simulink subsystem "Day3_Scenario_2"  (R2024a)
settings: Solver=VariableStepAuto  StartTime=0.0  StopTime=10.0  RelTol=1e-3
libraries: CarMaker4SL x8, slpidlib x1
settings Model: Creator=junhyung.cha  LastModifiedBy=User

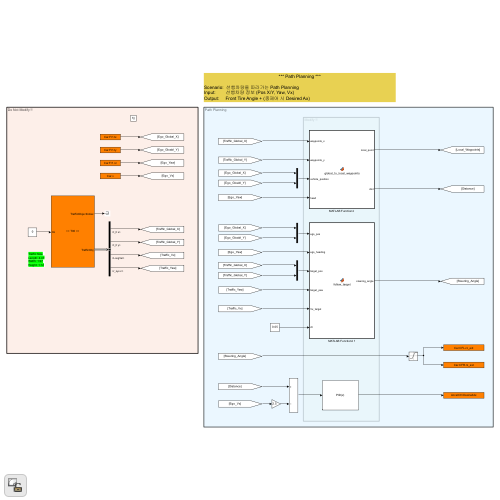
[thumbnail: Simulink's stored preview of the top-level diagram]
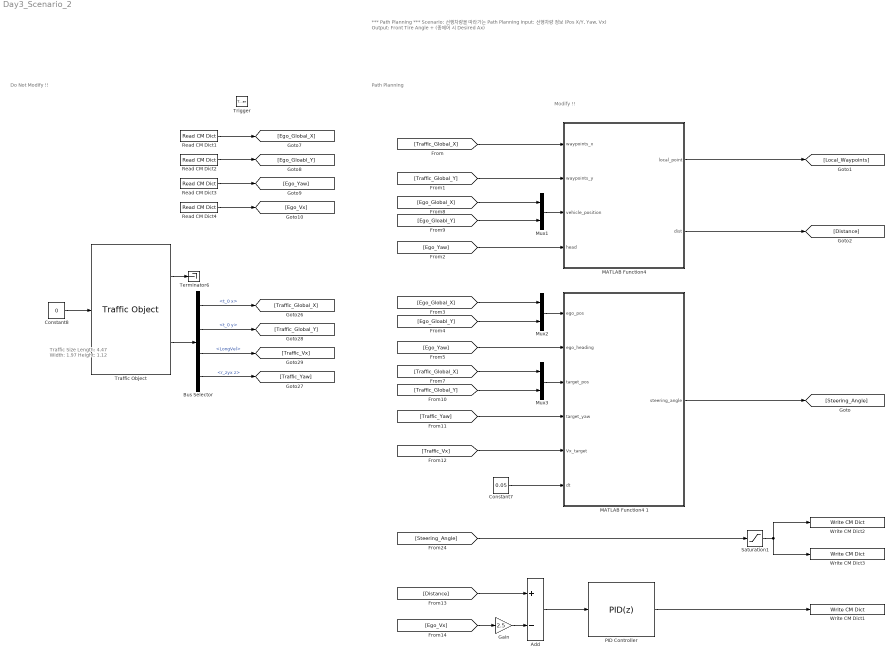
== system Day3_Scenario_2 ==
  note: Path Planning
  note: Do Not Modify !!
  note: Modify !!
  note: *** Path Planning ***
      |
      | Scenario: 선행차량을 따라가는 Path Planning
      | Input: 선행차량 정보 (Pos X/Y, Yaw, Vx)
      | Output: Front Tire Angle + (종제어 시 Desired Ax)
  note: Traffic Size
      | Length: 4.47
      | Width: 1.97
      | Height: 1.12
  Trigger : TriggerPort  TriggerType=function-call  VariantControl=(inherit)
  Add : Sum  Inputs=+-
  Bus Selector : BusSelector  OutputSignals=t_0 x,t_0 y,LongVel,r_zyx z
  Constant7 : Constant  Value=0.05
  Constant8 : Constant  Value=0
  Gain : Gain  Gain=2.5
  "MATLAB Function4 " : MATLAB Function  TreatAsAtomicUnit=on
  MATLAB Function4 1 : MATLAB Function  TreatAsAtomicUnit=on
  Mux1 : Mux  Inputs=2
  Mux2 : Mux  Inputs=2
  Mux3 : Mux  Inputs=2
  PID Controller : slpidlib/PID Controller  Controller=PID  Form=Parallel  TimeDomain=Discrete-time  UseExternalTs=off  SampleTime=-1  IntegratorMethod=Forward Euler  FilterMethod=Forward Euler  ControllerParametersSource=internal  P=3  I=0.01  UseKiTs=off  D=0  UseExternalDerivativeSource=off  N=100  UseFilter=on  TunerSelectOption=Transfer Function Based (PID Tuner App)  InitialConditionSource=internal  InitialConditionForIntegrator=0  InitialConditionForFilter=0  DifferentiatorICPrevScaledInput=0  ExternalReset=none  TrackingMode=off  Kt=1  LimitOutput=off  SatLimitsSource=internal  UpperSaturationLimit=inf  LowerSaturationLimit=-inf  LinearizeAsGain=on  AntiWindupMode=none  Kb=1  LimitIntegrator=off  UpperIntegratorSaturationLimit=inf  LowerIntegratorSaturationLimit=-inf  POutMin=[]  POutMax=[]  IOutMin=[]  IOutMax=[]  DOutMin=[]  DOutMax=[]  NOutMin=[]  NOutMax=[]  SumOutMin=[]  SumOutMax=[]  SaturationOutMin=[]  SaturationOutMax=[]  PParamMin=[]  PParamMax=[]  IParamMin=[]  IParamMax=[]  DParamMin=[]  DParamMax=[]  NParamMin=[]  NParamMax=[]  KbParamMin=[]  KbParamMax=[]  KtParamMin=[]  KtParamMax=[]  KbOutMin=[]  KbOutMax=[]  KtOutMin=[]  KtOutMax=[]  IntegratorOutMin=[]  IntegratorOutMax=[]  FilterOutMin=[]  FilterOutMax=[]  SumI1OutMin=[]  SumI1OutMax=[]  SumI2OutMin=[]  SumI2OutMax=[]  SumI3OutMin=[]  SumI3OutMax=[]  SumI4OutMin=[]  SumI4OutMax=[]  SumDOutMin=[]  SumDOutMax=[]  DifferentiatorOutMin=[]  DifferentiatorOutMax=[]  FilterDiffOutCoefMin=[]  FilterDiffOutCoefMax=[]  ReciprocalOutMin=[]  ReciprocalOutMax=[]  SumDenOutMin=[]  SumDenOutMax=[]  SumNumOutMin=[]  SumNumOutMax=[]  DivideOutMin=[]  DivideOutMax=[]  UdiffTsProdOutMin=[]  UdiffTsProdOutMax=[]  NTsProdOutMin=[]  NTsProdOutMax=[]  UintegralTsProdOutMin=[]  UintegralTsProdOutMax=[]  UngainTsProdOutMin=[]  UngainTsProdOutMax=[]  ClampingZeroOutDataTypeStr=Inherit: Inherit via back propagation  ClampingZeroOutMin=[]  ClampingZeroOutMax=[]  FilterDenConstantOutDataTypeStr=Inherit: Inherit via back propagation  FilterDenConstantOutMin=[]  FilterDenConstantOutMax=[]  PCopyOutDataTypeStr=Inherit: Inherit via back propagation  PCopyOutMin=[]  PCopyOutMax=[]  NCopyOutDataTypeStr=Inherit: Inherit via back propagation  NCopyOutMin=[]  NCopyOutMax=[]  IntegratorContinuousStateAttributes=''  IntegratorStateMustResolveToSignalObject=off  IntegratorRTWStateStorageClass=Auto  FilterContinuousStateAttributes=''  FilterStateMustResolveToSignalObject=off  FilterRTWStateStorageClass=Auto  ParallelPVariant=InternalParameters  IdealPVariant=Disabled  IVariant=InternalParameters  DVariant=InternalParameters  IntegratorVariant=Discrete  SatVariant=Disabled  AWVariant=Passthrough  PCopyVariant=Disabled  TRVariant=Disabled  FdbkBlocksVariant=Forward  IdealPFdbkVariant=Disabled  SatFdbkVariant=Disabled  DerivativeFilterVariant=ForwardEulerFilter  NVariant=InternalParameters  NCopyVariant=Disabled  FilterICVariant=InternalICsFilter  IntegratorICVariant=InternalICs  ExternalResetVariant=Disabled  TRSumVariant=Passthrough  SumFdbkVariant=Disabled  SumVariant=Sum_PID  TsampFilterVariant=InternalTs  TsampNgainVariant=Passthrough  TsampIntegralVariant=Disabled_SignalSpec  ExternalSaturationOutDataTypeStr=Inherit: Same as second input  DerivativeSourceVariant=ErrorSignal
  Read CM Dict1 : CarMaker4SL/Read CM Dict  xname=Car.Fr1.tx  xsync=off  xstime=Inherited
  Read CM Dict2 : CarMaker4SL/Read CM Dict  xname=Car.Fr1.ty  xsync=off  xstime=Inherited
  Read CM Dict3 : CarMaker4SL/Read CM Dict  xname=Car.Fr1.rz  xsync=off  xstime=Inherited
  Read CM Dict4 : CarMaker4SL/Read CM Dict  xname=Car.v  xsync=off  xstime=Inherited
  Saturation1 : Saturate  UpperLimit=pi/6  LowerLimit=-pi/6
  Terminator6 : Terminator
  Traffic Object : CarMaker4SL/Traffic Object  xname=T00  ximode=Traffic Id  xstime=Inherited
      settings: SourceProductName=CarMaker4SL
  Write CM Dict1 : CarMaker4SL/Write CM Dict  xname=AccelCtrl.DesiredAx  xsync=off
  Write CM Dict2 : CarMaker4SL/Write CM Dict  xname=Car.CFL.rz_ext  xsync=off
  Write CM Dict3 : CarMaker4SL/Write CM Dict  xname=Car.CFR.rz_ext  xsync=off
  wires:
  Read CM Dict4/1 -> [Ego_Vx]
  Saturation1/1 -> Write CM Dict3/1, Write CM Dict2/1
  Read CM Dict3/1 -> [Ego_Yaw]
  Read CM Dict1/1 -> [Ego_Global_X]
  Read CM Dict2/1 -> [Ego_Gloabl_Y]
  [Steering_Angle] -> Saturation1/1
  Traffic Object/2 -> Bus Selector/1
  Constant8/1 -> Traffic Object/1
  Bus Selector/4 -> [Traffic_Yaw]  "<r_zyx z>"
  Bus Selector/3 -> [Traffic_Vx]  "<LongVel>"
  Traffic Object/1 -> Terminator6/1
  Bus Selector/2 -> [Traffic_Global_Y]  "<t_0 y>"
  Bus Selector/1 -> [Traffic_Global_X]  "<t_0 x>"
  [Traffic_Global_X] -> "MATLAB Function4 "/1(waypoints_x)
  [Traffic_Global_Y] -> "MATLAB Function4 "/2(waypoints_y)
  [Ego_Gloabl_Y] -> Mux1/2
  Mux1/1 -> "MATLAB Function4 "/3(vehicle_position)
  [Ego_Global_X] -> Mux1/1
  [Ego_Yaw] -> "MATLAB Function4 "/4(head)
  "MATLAB Function4 "/1(local_point) -> [Local_Waypoints]
  "MATLAB Function4 "/2(dist) -> [Distance]
  [Ego_Global_X] -> Mux2/1
  [Ego_Gloabl_Y] -> Mux2/2
  Mux2/1 -> MATLAB Function4 1/1(ego_pos)
  [Ego_Yaw] -> MATLAB Function4 1/2(ego_heading)
  [Traffic_Global_X] -> Mux3/1
  [Traffic_Global_Y] -> Mux3/2
  [Traffic_Yaw] -> MATLAB Function4 1/4(target_yaw)
  Mux3/1 -> MATLAB Function4 1/3(target_pos)
  [Traffic_Vx] -> MATLAB Function4 1/5(Vx_target)
  Constant7/1 -> MATLAB Function4 1/6(dt)
  MATLAB Function4 1/1(steering_angle) -> [Steering_Angle]
  [Distance] -> Add/1
  [Ego_Vx] -> Gain/1
  Add/1 -> PID Controller/1
  PID Controller/1 -> Write CM Dict1/1
  Gain/1 -> Add/2

== matlab function Day3_Scenario_2/MATLAB Function4  ==
  settings: sampleTime=0.1
  data: waypoints_x input; waypoints_y input; local_point output; vehicle_position input; head input; dist output
function [local_point, dist] = global_to_local_waypoints(waypoints_x, waypoints_y, vehicle_position, head)

% Input
% waypoints_x       : Target vehicle global X [m]
% waypoints_y       : Target vehicle global Y [m]
% vehicle_position  : [Ego_Global_X; Ego_Global_Y]
% head              : Ego yaw [rad]
%
% Output
% local_point       : target position in ego local frame [x_local; y_local]
% dist              : distance between ego and target [m]

ego_x = vehicle_position(1);
ego_y = vehicle_position(2);
ego_yaw = head;

target_x = waypoints_x;
target_y = waypoints_y;

dx = target_x - ego_x;
dy = target_y - ego_y;

% Global → Ego Local 좌표 변환
x_local =  cos(ego_yaw) * dx + sin(ego_yaw) * dy;
y_local = -sin(ego_yaw) * dx + cos(ego_yaw) * dy;

local_point = [x_local; y_local];

dist = sqrt(dx^2 + dy^2);

end

== matlab function Day3_Scenario_2/MATLAB Function4 1 ==
  settings: sampleTime=0.1
  data: ego_pos input; ego_heading input; steering_angle output; target_pos input; target_yaw input; Vx_target input; dt input
function steering_angle = follow_target(ego_pos, ego_heading, target_pos, target_yaw, Vx_target, dt)

% Input
% ego_pos      : [Ego_Global_X; Ego_Global_Y]
% ego_heading  : Ego yaw [rad]
% target_pos   : [Traffic_Global_X; Traffic_Global_Y]
% target_yaw   : Traffic yaw [rad]
% Vx_target    : Target vehicle longitudinal velocity [m/s]
% dt           : sample time [s]
%
% Output
% steering_angle : front tire steering angle [rad]

% 차량 파라미터
L = 2.7;   % wheelbase [m]

% 선행차량 위치
ego_x = ego_pos(1);
ego_y = ego_pos(2);

tar_x = target_pos(1);
tar_y = target_pos(2);

% 선행차량 위치를 조금 예측
predict_time = 0.3;   % [s]
tar_x_pred = tar_x + Vx_target * predict_time * cos(target_yaw);
tar_y_pred = tar_y + Vx_target * predict_time * sin(target_yaw);

% Ego 기준 상대 위치
dx = tar_x_pred - ego_x;
dy = tar_y_pred - ego_y;

% Global → Ego Local 변환
x_local =  cos(ego_heading) * dx + sin(ego_heading) * dy;
y_local = -sin(ego_heading) * dx + cos(ego_heading) * dy;

% 선행차량이 너무 가까우면 조향이 튀므로 최소 lookahead 보정
Ld = sqrt(x_local^2 + y_local^2);

if Ld < 6
    Ld = 6;
elseif Ld > 30
    Ld = 30;
end

% 선행차량이 ego 뒤쪽으로 잡히면 조향 유지
persistent prev_steer

if isempty(prev_steer)
    prev_steer = 0;
end

if x_local < 1
    steering_cmd = prev_steer;
else
    % Pure Pursuit 기반 조향각
    alpha = atan2(y_local, x_local);
    steering_cmd = atan2(2 * L * sin(alpha), Ld);
end

% 조향각 제한
steer_max = 0.35;   % 약 20 deg

if steering_cmd > steer_max
    steering_cmd = steer_max;
elseif steering_cmd < -steer_max
    steering_cmd = -steer_max;
end

% 조향 변화율 제한
max_steer_rate = 0.8;   % rad/s
max_delta = max_steer_rate * dt;

delta = steering_cmd - prev_steer;

if delta > max_delta
    steering_angle = prev_steer + max_delta;
elseif delta < -max_delta
    steering_angle = prev_steer - max_delta;
else
    steering_angle = steering_cmd;
end

prev_steer = steering_angle;

end
